simulink model "TP_FWFCR_RL_Load"  (R2024b)
settings: Solver=VariableStepAuto  StartTime=0.0  StopTime=0.2  RelTol=1e-3
InitFcn:
  | a=30
  | pw=33.33
libraries: spsThyristorLib x6, spsSeriesRLCBranchLib x1, spsThreePhaseVIMeasurementLib x1, spsThreePhaseSourceLib x1, spsVoltageMeasurementLib x1, sps_lib x1
settings Model: Creator=admin  LastModifiedBy=admin

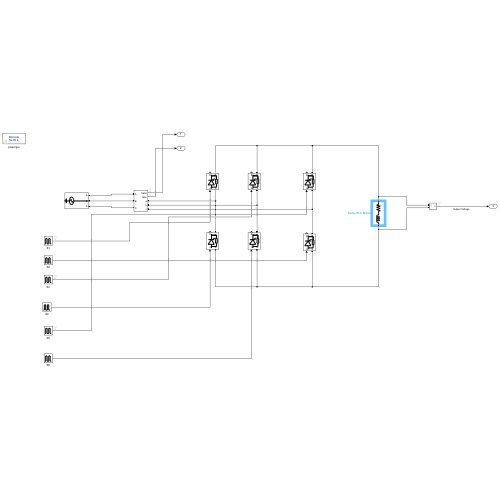
[thumbnail: Simulink's stored preview of the top-level diagram]
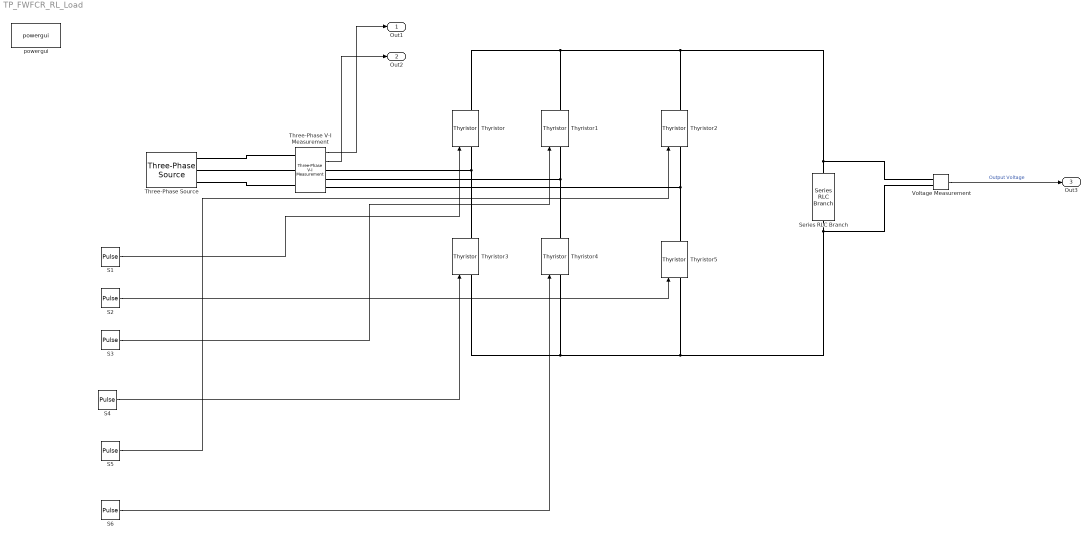
== system TP_FWFCR_RL_Load ==
  S1 : DiscretePulseGenerator  PulseType=Time based  Period=0.02  PulseWidth=pw  PhaseDelay=a*(0.02/360)
  S2 : DiscretePulseGenerator  PulseType=Time based  Period=0.02  PulseWidth=pw  PhaseDelay=(a+60)*(0.02/360)
  S3 : DiscretePulseGenerator  PulseType=Time based  Period=0.02  PulseWidth=pw  PhaseDelay=(a+120)*(0.02/360)
  S4 : DiscretePulseGenerator  PulseType=Time based  Period=0.02  PulseWidth=pw  PhaseDelay=(a+180)*(0.02/360)
  S5 : DiscretePulseGenerator  PulseType=Time based  Period=0.02  PulseWidth=pw  PhaseDelay=(a+240)*(0.02/360)
  S6 : DiscretePulseGenerator  PulseType=Time based  Period=0.02  PulseWidth=pw  PhaseDelay=(a+300)*(0.02/360)
  Series RLC Branch : spsSeriesRLCBranchLib/Series RLC Branch  LConnTagsString=__new0  RConnTagsString=__new0  BranchType=RL  Resistance=5  Inductance=1  SetiL0=off  InitialCurrent=0  Capacitance=1e-6  Setx0=off  InitialVoltage=0  Measurements=None
  Three-Phase V-I Measurement : spsThreePhaseVIMeasurementLib/Three-Phase V-I Measurement  VoltageMeasurement=phase-to-phase  SetLabelV=off  LabelV=Vabc  Vpu=off  VpuLL=off  CurrentMeasurement=yes  SetLabelI=off  LabelI=Iabc  Ipu=off  Pbase=100e6  Vbase=500e3  OutputType=Complex  PhasorSimulation=off  PSBequivalent=0
  Three-Phase Source : spsThreePhaseSourceLib/Three-Phase Source  InternalConnection=Yg  VoltagePhases=off  Voltage=230  PhaseAngle=0  Voltage_phases=[25e3 25e3 25e3]/sqrt(3)  PhaseAngles_phases=[0 -120 +120]  Frequency=50  NonIdealSource=off  SpecifyImpedance=off  Resistance=0.8929  Inductance=16.58e-3  ShortCircuitLevel=100e6  BaseVoltage=25e3  XRratio=7  BusType=swing  Pref=10e3  Qref=0  Prefabc=[10e3, 10e3, 10e3]  Qrefabc=[0, 0, 0]  Qmin=-inf  Qmax=inf
  Thyristor{,1..5} (6 alike) : spsThyristorLib/Thyristor  Ron=0.001  Lon=0  Vf=0.8  IC=0  Rs=500  Cs=250e-9  Measurements=on
  Voltage Measurement : spsVoltageMeasurementLib/Voltage Measurement  PhasorSimulation=off  OutputType=Complex  PSBequivalent=0
  powergui : sps_lib/powergui  Priority=1  SimulationMode=Discrete  SampleTime=50e-6  frequency=60  Iterations=50  frequencyindice=50  Pbase=100e6  ErrMax=1e-4  UnitsV=kV  UnitsW=MW  buscounter=0  FunctionMessages=off  echomessages=off  EnableUseOfTLC=off  CurrentSourceSwitches=off  DisableSnubberDevices=off  DisableRonSwitches=off  DisableVfSwitches=off  DisplayEquations=off  AutomaticDiscreteSolvers=off  SolverType=Tustin/Backward Euler (TBE)  Interpol=off  ExternalGateDelay=off  methode=off  Ts=100  x0status=blocks  SPID=on  SwTol=0  HookPort=off  NonlinearTolerance=1e-4  nMaxIteration=100  ContinueOnMaxIteration=off  RestoreLinks=warning  ResistiveCurrentMeasurement=off  Frange=[0:2:500]  Ylog=off  Xlog=on  ShowGrid=off  save=off  variable=ZData  structure=0  ZoomFFT=off  StartTime=0.0  cycles=1  DisplayStyle=1  fundamental=60  FreqAxis=off  MaxFrequency=1000  frequencyindicesteady=1  RmsSteady=1  display=off
  Out1 : Outport
  Out2 : Outport  Port=2
  Out3 : Outport  Port=3
  wires:
  S1/1 -> Thyristor/1
  S2/1 -> Thyristor5/1
  S3/1 -> Thyristor1/1
  S4/1 -> Thyristor3/1
  S5/1 -> Thyristor2/1
  S6/1 -> Thyristor4/1
  Voltage Measurement/1 -> Out3/1  "Output Voltage"
  Three-Phase V-I Measurement/1 -> Out1/1
  Three-Phase V-I Measurement/2 -> Out2/1
  connections:
  Three-Phase Source/RConn1 -- Three-Phase V-I Measurement/LConn1
  Three-Phase Source/RConn2 -- Three-Phase V-I Measurement/LConn2
  Three-Phase Source/RConn3 -- Three-Phase V-I Measurement/LConn3
  Three-Phase V-I Measurement/RConn1 -- Thyristor/LConn1 -- Thyristor3/RConn1
  Three-Phase V-I Measurement/RConn2 -- Thyristor1/LConn1 -- Thyristor4/RConn1
  Three-Phase V-I Measurement/RConn3 -- Thyristor2/LConn1 -- Thyristor5/RConn1
  Thyristor3/LConn1 -- Voltage Measurement/LConn2 -- Series RLC Branch/RConn1 -- Thyristor5/LConn1 -- Thyristor4/LConn1
  Thyristor/RConn1 -- Voltage Measurement/LConn1 -- Series RLC Branch/LConn1 -- Thyristor2/RConn1 -- Thyristor1/RConn1
